simulink model "threephase_inverter_final"  (R2025a)
settings: Solver=ode23tb  StartTime=0.0  StopTime=0.2  RelTol=1e-3
model workspace (MAT data in the model file):
  x = 1
libraries: spsIGBTDiodeLib x6, spsGroundLib x3, spsSeriesRLCBranchLib x3, spsSeriesRLCLoadLib x3, dspstat3 x2, spsDCVoltageSourceLib x1, spsThreePhaseSeriesRLCBranchLib x1, spsThreePhaseSeriesRLCLoadLib x1, spsThreePhaseVIMeasurementLib x1, spsTriangleGeneratorLib x1, spsVoltageMeasurementLib x1, spspowerguiLib x1
settings Model: Creator=asus  LastModifiedBy=asus

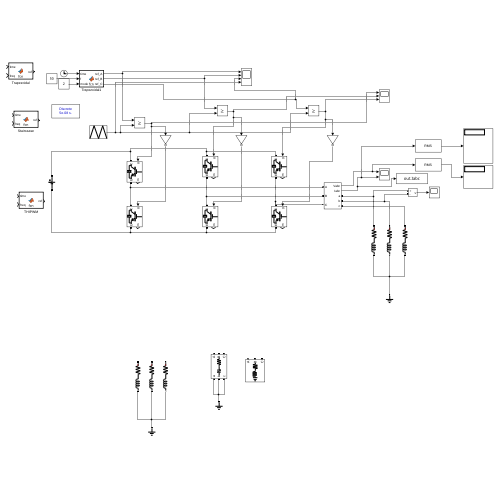
[thumbnail: Simulink's stored preview of the top-level diagram]
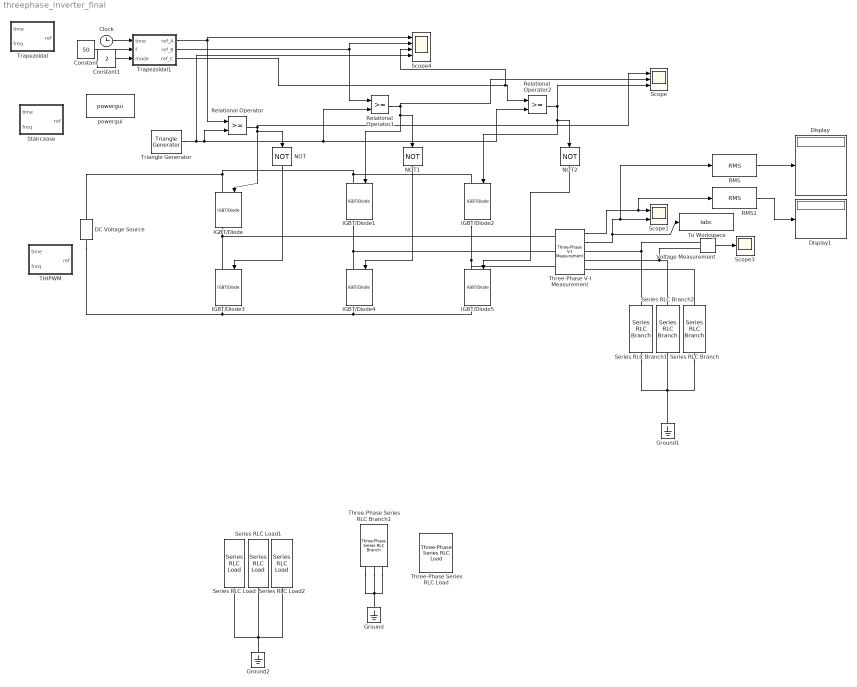
== system threephase_inverter_final ==
  Clock : Clock
  Constant : Constant  Value=50
  Constant1 : Constant  Value=2
  DC Voltage Source : spsDCVoltageSourceLib/DC Voltage Source  Amplitude=100  Measurements=None
  Display : Display
  Display1 : Display
  Ground : spsGroundLib/Ground  LConnTagsString=a
  Ground1 : spsGroundLib/Ground  LConnTagsString=a
  Ground2 : spsGroundLib/Ground  LConnTagsString=a
  IGBT/Diode{,1..5} (6 alike) : spsIGBTDiodeLib/IGBT//Diode  Ron=1e-3  Rs=1e5  Cs=inf  Measurements=on
  NOT : Logic  Operator=NOT  IconShape=distinctive  AllPortsSameDT=off  OutDataTypeStr=boolean
  NOT1 : Logic  Operator=NOT  IconShape=distinctive  AllPortsSameDT=off  OutDataTypeStr=boolean
  NOT2 : Logic  Operator=NOT  IconShape=distinctive  AllPortsSameDT=off  OutDataTypeStr=boolean
  RMS : dspstat3/RMS  run=off  directionMode=Each column  dimension=1  reset_popup=None
  RMS1 : dspstat3/RMS  run=off  directionMode=Each column  dimension=1  reset_popup=None
  Relational Operator : RelationalOperator  OutDataTypeStr=boolean  RndMeth=Simplest  InputSameDT=off
  Relational Operator1 : RelationalOperator  OutDataTypeStr=boolean  RndMeth=Simplest  InputSameDT=off
  Relational Operator2 : RelationalOperator  OutDataTypeStr=boolean  RndMeth=Simplest  InputSameDT=off
  Scope : Scope  NumInputPorts=3
      settings: ActiveDisplayYMinimum=-0.11975341028331582  ActiveDisplayYMaximum=1.1302465897166842
  Scope1 : Scope  NumInputPorts=2
      settings: ActiveDisplayYMinimum=-121.19748956159052  ActiveDisplayYMaximum=116.89773997839771
  Scope3 : Scope
      settings: ActiveDisplayYMinimum=-125.19432061008159  ActiveDisplayYMaximum=125.0398681567131  DataLoggingVariableName=ScopeData3
  Scope4 : Scope  NumInputPorts=4
      settings: ActiveDisplayYMinimum=-1.25  ActiveDisplayYMaximum=1.25  DataLoggingVariableName=ScopeData4
  Series RLC Branch : spsSeriesRLCBranchLib/Series RLC Branch  LConnTagsString=__new0  RConnTagsString=__new0  BranchType=RL  Resistance=100  Inductance=50e-3  SetiL0=off  InitialCurrent=0  Capacitance=0  Setx0=off  InitialVoltage=0  Measurements=None
  Series RLC Branch1 : spsSeriesRLCBranchLib/Series RLC Branch  LConnTagsString=__new0  RConnTagsString=__new0  BranchType=RL  Resistance=100  Inductance=50e-3  SetiL0=off  InitialCurrent=0  Capacitance=0  Setx0=off  InitialVoltage=0  Measurements=None
  Series RLC Branch2 : spsSeriesRLCBranchLib/Series RLC Branch  LConnTagsString=__new0  RConnTagsString=__new0  BranchType=RL  Resistance=100  Inductance=50e-3  SetiL0=off  InitialCurrent=0  Capacitance=0  Setx0=off  InitialVoltage=0  Measurements=None
  Series RLC Load : spsSeriesRLCLoadLib/Series RLC Load  LConnTagsString=a  RConnTagsString=__new0  NominalVoltage=1000  NominalFrequency=50  ActivePower=1e3  InductivePower=5e3  CapacitivePower=0  Setx0=off  InitialVoltage=0  SetiL0=off  InitialCurrent=0  Measurements=None  LoadType=constant Z
  Series RLC Load1 : spsSeriesRLCLoadLib/Series RLC Load  LConnTagsString=a  RConnTagsString=__new0  NominalVoltage=1000  NominalFrequency=50  ActivePower=1e3  InductivePower=5e3  CapacitivePower=0  Setx0=off  InitialVoltage=0  SetiL0=off  InitialCurrent=0  Measurements=None  LoadType=constant Z
  Series RLC Load2 : spsSeriesRLCLoadLib/Series RLC Load  LConnTagsString=a  RConnTagsString=__new0  NominalVoltage=1000  NominalFrequency=50  ActivePower=1e3  InductivePower=5e3  CapacitivePower=0  Setx0=off  InitialVoltage=0  SetiL0=off  InitialCurrent=0  Measurements=None  LoadType=constant Z
  Staircaase : MATLAB Function  TreatAsAtomicUnit=on
  THIPWM : MATLAB Function  TreatAsAtomicUnit=on
  Three-Phase Series RLC Branch1 : spsThreePhaseSeriesRLCBranchLib/Three-Phase Series RLC Branch  LConnTagsString=A|B|C  RConnTagsString=A|B|C  BranchType=RC  Resistance=100  Inductance=1e-3  Capacitance=20e-5  Measurements=None
  Three-Phase Series RLC Load : spsThreePhaseSeriesRLCLoadLib/Three-Phase Series RLC Load  LConnTagsString=A|B|C  Configuration=Y (grounded)  NominalVoltage=1000  Vabc=[1e3 1e3 1e3]  Vabcp=[1e3 1e3 1e3]  NominalFrequency=50  UnbalancedPower=off  ActivePower=1e3  InductivePower=5e3  CapacitivePower=0  Pabc=[10e3 9e3 11e3]  QLabc=[100 90 110]  QCabc=[100 90 110]  Pabcp=[10e3 9e3 11e3]  QLabcp=[100 90 110]  QCabcp=[100 90 110]  Measurements=None  LoadType=constant Z
  Three-Phase V-I Measurement : spsThreePhaseVIMeasurementLib/Three-Phase V-I Measurement  VoltageMeasurement=phase-to-phase  SetLabelV=off  LabelV=Vabc  Vpu=off  VpuLL=off  CurrentMeasurement=yes  SetLabelI=off  LabelI=Iabc  Ipu=off  Pbase=100e6  Vbase=500e3  OutputType=Complex  PhasorSimulation=off  PSBequivalent=0
  To Workspace : ToWorkspace  VariableName=Iabc  SaveFormat=Structure With Time  SampleTime=-1
      settings: MaxDataPoints=10000
  Trapezoidal : MATLAB Function  TreatAsAtomicUnit=on
  Trapezoidal1 : MATLAB Function  TreatAsAtomicUnit=on
  Triangle Generator : spsTriangleGeneratorLib/Triangle Generator  Freq=5e3  Phase=0  Ts=0
  Voltage Measurement : spsVoltageMeasurementLib/Voltage Measurement  PhasorSimulation=off  OutputType=Complex  PSBequivalent=0
  powergui : spspowerguiLib/powergui  Priority=1  SimulationMode=Discrete  SampleTime=5e-8  frequency=60  Iterations=50  frequencyindice=0  Pbase=100e6  ErrMax=1e-4  UnitsV=kV  UnitsW=MW  buscounter=0  FunctionMessages=off  echomessages=off  EnableUseOfTLC=off  CurrentSourceSwitches=off  DisableSnubberDevices=off  DisableRonSwitches=off  DisableVfSwitches=off  DisplayEquations=off  AutomaticDiscreteSolvers=off  SolverType=Tustin/Backward Euler (TBE)  Interpol=off  ExternalGateDelay=off  methode=off  Ts=100  x0status=blocks  SPID=on  SwTol=0  HookPort=off  NonlinearTolerance=1e-4  nMaxIteration=100  ContinueOnMaxIteration=off  RestoreLinks=warning  ResistiveCurrentMeasurement=off  Frange=[0:2:500]  Ylog=off  Xlog=on  ShowGrid=off  save=off  variable=ZData  structure=0  ZoomFFT=off  StartTime=0.0  cycles=1  DisplayStyle=1  fundamental=60  FreqAxis=off  MaxFrequency=1000  frequencyindicesteady=1  RmsSteady=1  display=off
  wires:
  Trapezoidal1/1(ref_A) -> Relational Operator/1, Scope4/1
  Three-Phase V-I Measurement/1 -> RMS1/1, Scope1/1
  Trapezoidal1/2(ref_B) -> Relational Operator1/1, Scope4/2
  Relational Operator1/1 -> Scope/2, IGBT/Diode1/1, NOT1/1
  Trapezoidal1/3(ref_C) -> Scope4/3, Relational Operator2/1
  Triangle Generator/1 -> Scope4/4, Relational Operator2/2, Relational Operator1/2, Relational Operator/2
  Relational Operator2/1 -> Scope/3, IGBT/Diode2/1, NOT2/1
  Relational Operator/1 -> IGBT/Diode/1, NOT/1, Scope/1
  NOT/1 -> IGBT/Diode3/1
  NOT1/1 -> IGBT/Diode4/1
  NOT2/1 -> IGBT/Diode5/1
  Voltage Measurement/1 -> Scope3/1
  Three-Phase V-I Measurement/2 -> To Workspace/1, RMS/1, Scope1/2
  RMS/1 -> Display/1
  RMS1/1 -> Display1/1
  Clock/1 -> Trapezoidal1/1(time)
  Constant/1 -> Trapezoidal1/2(f)
  Constant1/1 -> Trapezoidal1/3(mode)
  connections:
  Three-Phase V-I Measurement/LConn1 -- IGBT/Diode3/LConn1 -- IGBT/Diode/RConn1
  Three-Phase V-I Measurement/LConn2 -- IGBT/Diode1/RConn1 -- IGBT/Diode4/LConn1
  Three-Phase V-I Measurement/LConn3 -- IGBT/Diode2/RConn1 -- IGBT/Diode5/LConn1
  DC Voltage Source/RConn1 -- IGBT/Diode2/LConn1 -- IGBT/Diode1/LConn1 -- IGBT/Diode/LConn1
  DC Voltage Source/LConn1 -- IGBT/Diode4/RConn1 -- IGBT/Diode5/RConn1 -- IGBT/Diode3/RConn1
  Voltage Measurement/LConn1 -- Series RLC Branch1/LConn1 -- Three-Phase V-I Measurement/RConn1
  Voltage Measurement/LConn2 -- Series RLC Branch2/LConn1 -- Three-Phase V-I Measurement/RConn2
  Series RLC Branch/LConn1 -- Three-Phase V-I Measurement/RConn3
  Three-Phase Series RLC Branch1/RConn2 -- Three-Phase Series RLC Branch1/RConn1 -- Three-Phase Series RLC Branch1/RConn3 -- Ground/LConn1
  Ground1/LConn1 -- Series RLC Branch/RConn1 -- Series RLC Branch2/RConn1 -- Series RLC Branch1/RConn1
  Ground2/LConn1 -- Series RLC Load2/RConn1 -- Series RLC Load/RConn1 -- Series RLC Load1/RConn1

== matlab function threephase_inverter_final/THIPWM ==
  data: time input; ref output; freq input
function ref = fcn(time, freq)
    theta = 2*pi*freq*time;
    Vf = sin(theta) + (1/6) * sin(3*theta); % Fundamental + 3rd harmonic
    % Normalize so peak = 1
    ref = Vf / 1.15; 
end

== matlab function threephase_inverter_final/Trapezoidal ==
  data: time input; ref output; freq input
function ref = fcn(time, freq)
    tr = sawtooth(2*pi*freq*time, 0.5); % Standard triangle
    % Clip the triangle to create a trapezoid
    t_flat = max(-0.85, min(0.85, tr)); % Clip at 0.85 (approximation)
    ref = t_flat; 
end

== matlab function threephase_inverter_final/Staircaase ==
  data: time input; ref output; freq input
function ref = fcn(time, freq)
    raw_sine = sin(2*pi*freq*time);
    num_steps = 7; % Number of voltage steps per half cycle
    % Quantize the sine wave
    ref = round(raw_sine * num_steps) / num_steps;
end

== matlab function threephase_inverter_final/Trapezoidal1 ==
  data: time input; ref_A output; f input; mode input; ref_B output; ref_C output
function [ref_A, ref_B, ref_C] = fcn(time, f, mode)
    omega = 2*pi*f;
    theta = omega * time;
    num_steps = 7; % Number of steps for Staircase (7 or 9 typical)
    
    % Phase Angle Calculation (Separated by 120 degrees)
    theta_A = theta;
    theta_B = theta - 2*pi/3;
    theta_C = theta + 2*pi/3; 
    
    % Generate the specific waveform for each phase
    ref_A = generate_waveform(theta_A, mode, num_steps);
    ref_B = generate_waveform(theta_B, mode, num_steps);
    ref_C = generate_waveform(theta_C, mode, num_steps);
end

function y = generate_waveform(theta, mode, num_steps)
    switch mode
        case 1 % Standard Sinusoidal PWM (For comparison)
            y = sin(theta);
            
        case 2 % Trapezoidal Modulation
            % Use sawtooth to get a triangle, then clip it for the trapezoid
            tri = sawtooth(theta, 0.5); 
            % Clip at 0.85 to get the flat top of the trapezoid
            y = max(-0.85, min(0.85, tri)); 

        case 3 % Staircase Modulation
            % Round the sine wave to discrete steps
            y = round(sin(theta) * num_steps) / num_steps;

        case 4 % 3rd Harmonic Injected PWM (THIPWM)
            % Fundamental + 1/6th of 3rd harmonic
            V_thi = sin(theta) + (1/6)*sin(3*theta);
            % CRITICAL: Normalize to 1.0 peak so it compares correctly with the carrier
            y = V_thi / 1.15; 
            
        otherwise
            y = sin(theta);
    end
end
